simulink model "gm_sampleModel1956_3_sub_sub_sub"  (R2023a)
settings: Solver=VariableStepAuto  StartTime=0.0  StopTime=10.0  RelTol=1e-3
libraries: hdlsllib x4, simulink x3
settings Model: Creator=user1  LastModifiedBy=user1
settings OptimizationCC: BlockReduction=off  ConditionallyExecuteInputs=off
settings DebuggingCC: InheritedTsInSrcMsg=none

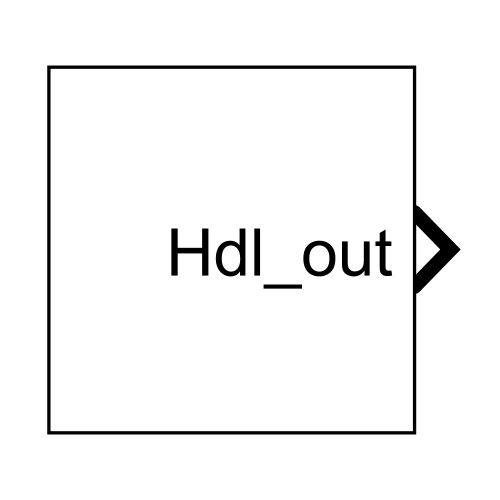
[thumbnail: Simulink's stored preview of the top-level diagram]
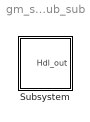
== system gm_sampleModel1956_3_sub_sub_sub ==
  Subsystem : Subsystem

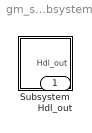
== system gm_sampleModel1956_3_sub_sub_sub/Subsystem ==
  Subsystem : Subsystem
  Hdl_out : Outport  OutDataTypeStr=uint8

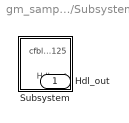
== system gm_sampleModel1956_3_sub_sub_sub/Subsystem/Subsystem ==
  Subsystem : Subsystem
  Hdl_out : Outport  OutDataTypeStr=uint8

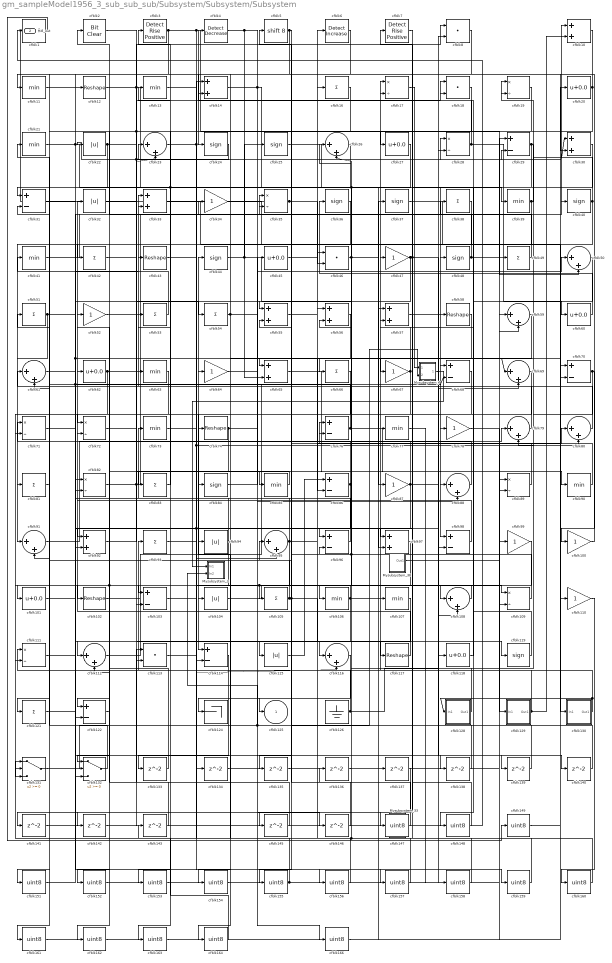
== system gm_sampleModel1956_3_sub_sub_sub/Subsystem/Subsystem/Subsystem ==
  Mysubsystem_3 : Subsystem  TreatAsAtomicUnit=on  RTWFcnName=Mysubsystem_3
      settings: RTWFcnNameOpts=User specified  RTWFileNameOpts=Use function name
  Mysubsystem_33 : Subsystem  TreatAsAtomicUnit=on  RTWFcnName=Mysubsystem_33
      settings: RTWFcnNameOpts=User specified  RTWFileNameOpts=Use function name
  Mysubsystem_38 : Subsystem  TreatAsAtomicUnit=on  RTWFcnName=Mysubsystem_38
      settings: RTWFcnNameOpts=User specified  RTWFileNameOpts=Use function name
  Mysubsystem_7 : Subsystem  TreatAsAtomicUnit=on  RTWFcnName=Mysubsystem_7
      settings: RTWFcnNameOpts=User specified  RTWFileNameOpts=Use function name
  cfblk1 : hdlsllib/Logic and Bit Operations/Compare To Zero  relop=<=  OutDataTypeStr=uint8
  cfblk{10,14,30,33,55..57,65,92,97} (10 alike) : Sum  OutDataTypeStr=uint8
  cfblk{34,47,52,64,67,78,87,99..100,110} (10 alike) : Gain  OutDataTypeStr=uint8
  cfblk{20,27,45,60,62,101,118} (7 alike) : Bias  Bias=0.0  SaturateOnIntegerOverflow=off
  cfblk{12,43,58,74,102,117} (6 alike) : Reshape
  cfblk{29,31,68,70,76,86,96,98,103,114,122} (11 alike) : Sum  Inputs=+-  OutDataTypeStr=uint8
  cfblk{22,32,94,104,115} (5 alike) : Abs  OutDataTypeStr=uint8  SaturateOnIntegerOverflow=off
  cfblk{16,38,42,49,51,53..54,66,81,83,93,105,121} (13 alike) : Sum  Inputs=+  OutDataTypeStr=uint8
  cfblk{11,13,21,39,41,63,73,77,85,90,106..107} (12 alike) : MinMax  OutDataTypeStr=uint8
  cfblk{23,26,50,59,61,69,79..80,88,91,95,108,112,116} (14 alike) : Sum  Inputs=|++  OutDataTypeStr=uint8
  cfblk{17,19,28,35,71..72,82,89,109,111} (10 alike) : Product  Inputs=*/  OutDataTypeStr=uint8  RndMeth=Zero  SaturateOnIntegerOverflow=on
  cfblk{8,18,46,113} (4 alike) : DotProduct  OutDataTypeStr=uint8
  cfblk{24..25,36..37,40,44,48,84,119} (9 alike) : Signum
  cfblk124 : Terminator
  cfblk126 : Ground
  cfblk128 : Subsystem
      settings: LibrarySourceBlock=|
      | hdlsllib/Ports &
      | Subsystems/Subsystem
  cfblk129 : Subsystem
      settings: LibrarySourceBlock=|
      | hdlsllib/Ports &
      | Subsystems/Subsystem
  cfblk130 : Subsystem
      settings: LibrarySourceBlock=|
      | hdlsllib/Ports &
      | Subsystems/Subsystem
  cfblk131 : Switch  OutDataTypeStr=uint8  SaturateOnIntegerOverflow=off  InputSameDT=off
  cfblk132 : Switch  OutDataTypeStr=uint8  SaturateOnIntegerOverflow=off  InputSameDT=off
  cfblk{133..143,145..146} (13 alike) : Delay  SampleTime=1
  cfblk{147..149,151..164,166} (18 alike) : DataTypeConversion  OutDataTypeStr=uint8  SaturateOnIntegerOverflow=off  RndMeth=Floor
  cfblk2 : simulink/Logic and Bit Operations/Bit Clear  iBit=0
      settings: LibrarySourceBlock=|
      | hdlsllib/Logic and Bit
      | Operations/Bit Clear
  cfblk3 : hdlsllib/Logic and Bit Operations/Detect Rise Positive  vinit=0  OutDataTypeStr=uint8
  cfblk4 : simulink/Logic and Bit Operations/Detect Decrease  vinit=0.0  OutDataTypeStr=uint8
      settings: LibrarySourceBlock=|
      | hdlsllib/Logic and Bit
      | Operations/Detect
      | Decrease
  cfblk5 : ArithShift  BitShiftNumber=8
  cfblk6 : simulink/Logic and Bit Operations/Detect Increase  vinit=0.0  OutDataTypeStr=uint8
      settings: LibrarySourceBlock=|
      | hdlsllib/Logic and Bit
      | Operations/Detect
      | Increase
  cfblk7 : hdlsllib/Logic and Bit Operations/Detect Rise Positive  vinit=0  OutDataTypeStr=uint8
  cfblk125 : Outport  OutDataTypeStr=uint8  VectorParamsAs1DForOutWhenUnconnected=off
  Hdl_out : Outport  Port=2  OutDataTypeStr=uint8
  wires:
  Mysubsystem_38/1(Out1) -> cfblk59/1
  Mysubsystem_33/1(Out1) -> cfblk1/1
  cfblk42/1 -> Mysubsystem_33/1(In1)
  Mysubsystem_7/1(Out1) -> Mysubsystem_3/1(In1)
  cfblk17/1 -> Mysubsystem_7/1(In1)
  cfblk166/1 -> cfblk59/2
  cfblk64/1 -> cfblk166/1
  cfblk164/1 -> cfblk143/1
  cfblk59/1 -> cfblk164/1
  cfblk163/1 -> cfblk99/1
  cfblk162/1 -> cfblk57/1
  cfblk99/1 -> cfblk162/1
  cfblk161/1 -> cfblk110/1
  cfblk160/1 -> cfblk94/1, cfblk26/1
  cfblk159/1 -> cfblk77/1
  cfblk13/1 -> cfblk159/1
  cfblk158/1 -> cfblk136/1, cfblk14/1
  cfblk157/1 -> cfblk56/2
  cfblk93/1 -> cfblk157/1
  cfblk156/1 -> cfblk56/1
  cfblk101/1 -> cfblk156/1
  cfblk155/1 -> cfblk131/1, cfblk118/1
  cfblk154/1 -> cfblk107/1
  cfblk153/1 -> cfblk29/1
  cfblk107/1 -> cfblk153/1
  cfblk152/1 -> cfblk137/1
  cfblk19/1 -> cfblk152/1
  cfblk151/1 -> cfblk92/2
  cfblk137/1 -> cfblk151/1
  cfblk149/1 -> cfblk20/1
  cfblk1/1 -> cfblk149/1
  cfblk148/1 -> cfblk7/1
  cfblk147/1 -> cfblk5/1
  cfblk7/1 -> cfblk147/1
  cfblk146/1 -> cfblk95/1
  cfblk145/1 -> cfblk112/2
  cfblk143/1 -> cfblk113/1
  cfblk142/1 -> cfblk8/2
  cfblk141/1 -> cfblk46/1
  cfblk140/1 -> cfblk55/2
  cfblk139/1 -> cfblk96/2
  cfblk138/1 -> cfblk76/2
  cfblk136/1 -> cfblk108/2
  cfblk135/1 -> cfblk35/2
  cfblk134/1 -> cfblk89/1
  cfblk103/1 -> cfblk134/1
  cfblk133/1 -> cfblk82/1
  cfblk114/1 -> cfblk133/1
  cfblk11/1 -> cfblk12/1
  cfblk111/1 -> cfblk43/1
  cfblk45/1 -> cfblk38/1
  cfblk40/1 -> cfblk122/1, cfblk19/2
  cfblk5/1 -> cfblk125/1, cfblk61/2
  cfblk53/1 -> cfblk41/1
  cfblk77/1 -> cfblk158/1
  cfblk31/1 -> cfblk54/1
  cfblk29/1 -> cfblk67/1, cfblk79/2
  cfblk86/1 -> cfblk13/1, cfblk135/1
  cfblk16/1 -> cfblk112/1
  cfblk18/1 -> cfblk103/1
  cfblk105/1 -> cfblk117/1, cfblk145/1, cfblk51/1
  cfblk26/1 -> cfblk42/1
  cfblk10/1 -> cfblk30/2
  cfblk35/1 -> cfblk46/2, Hdl_out/1
  cfblk52/1 -> cfblk6/1
  cfblk73/1 -> cfblk109/2, cfblk105/1
  cfblk55/1 -> cfblk16/1
  cfblk113/1 -> cfblk95/2
  cfblk109/1 -> cfblk61/1, cfblk26/2
  cfblk56/1 -> cfblk155/1
  cfblk22/1 -> cfblk101/1, cfblk8/1
  cfblk102/1 -> cfblk84/1
  cfblk104/1 -> cfblk109/1
  cfblk8/1 -> cfblk27/1
  cfblk132/1 -> cfblk21/1
  cfblk122/1 -> cfblk52/1
  cfblk118/1 -> cfblk18/1
  cfblk72/1 -> cfblk17/2
  cfblk89/1 -> cfblk76/1
  cfblk97/1 -> cfblk141/1, cfblk142/1
  cfblk116/1 -> cfblk124/1
  cfblk85/1 -> cfblk83/1
  cfblk106/1 -> cfblk40/1, cfblk104/1, cfblk132/2
  cfblk83/1 -> cfblk23/1
  cfblk61/1 -> cfblk68/2, cfblk138/1
  cfblk20/1 -> cfblk113/2, cfblk31/1, cfblk11/1
  cfblk4/1 -> cfblk65/2, cfblk146/1
  cfblk81/1 -> cfblk121/1
  cfblk94/1 -> cfblk73/1, cfblk131/3
  cfblk39/1 -> cfblk19/1, cfblk148/1
  cfblk126/1 -> cfblk111/1, cfblk28/2
  cfblk23/1 -> cfblk119/1, cfblk18/2
  cfblk46/1 -> cfblk96/1, cfblk70/2
  cfblk119/1 -> cfblk57/2
  cfblk58/1 -> cfblk86/2
  cfblk50/1 -> cfblk78/1
  cfblk27/1 -> cfblk161/1, cfblk163/1, cfblk66/1
  cfblk76/1 -> cfblk90/1, cfblk31/2
  cfblk47/1 -> cfblk97/1, cfblk140/1, cfblk103/2
  cfblk128/1(Out1) -> cfblk64/1
  cfblk92/1 -> cfblk29/2
  cfblk57/1 -> cfblk58/1
  cfblk49/1 -> cfblk2/1
  cfblk110/1 -> cfblk160/1
  cfblk74/1 -> cfblk92/1, cfblk88/2
  cfblk32/1 -> cfblk30/1, cfblk14/2
  cfblk25/1 -> cfblk87/1
  cfblk54/1 -> cfblk50/1, cfblk154/1
  cfblk63/1 -> cfblk91/2
  cfblk34/1 -> cfblk130/1(In1)
  cfblk121/1 -> cfblk82/2
  cfblk30/1 -> cfblk68/1
  cfblk37/1 -> cfblk70/1
  cfblk78/1 -> cfblk129/1(In1)
  cfblk2/1 -> cfblk85/1
  cfblk80/1 -> cfblk63/1
  cfblk36/1 -> cfblk55/1
  cfblk12/1 -> cfblk48/1, cfblk23/2
  cfblk90/1 -> cfblk35/1
  cfblk6/1 -> cfblk74/1
  cfblk112/1 -> cfblk37/1
  cfblk48/1 -> cfblk3/1, cfblk50/2
  cfblk91/1 -> cfblk79/1
  cfblk84/1 -> cfblk45/1
  cfblk24/1 -> cfblk22/1
  cfblk71/1 -> cfblk34/1
  cfblk3/1 -> cfblk116/2, cfblk80/2, cfblk49/1, cfblk132/3
  cfblk98/1 -> cfblk72/2
  cfblk87/1 -> cfblk114/2, cfblk122/2, cfblk53/1, cfblk69/2
  cfblk66/1 -> cfblk71/2
  cfblk41/1 -> cfblk33/2
  cfblk82/1 -> cfblk10/1, cfblk28/1, cfblk115/1
  cfblk43/1 -> cfblk89/2
  cfblk14/1 -> cfblk39/1, cfblk139/1
  cfblk33/1 -> cfblk88/1
  cfblk62/1 -> cfblk65/1, cfblk131/2
  cfblk95/1 -> cfblk62/1, cfblk111/2, cfblk80/1
  cfblk88/1 -> cfblk71/1
  cfblk69/1 -> cfblk72/1
  cfblk100/1 -> cfblk24/1
  cfblk108/1 -> cfblk102/1
  cfblk68/1 -> cfblk114/1
  cfblk96/1 -> cfblk44/1
  cfblk60/1 -> cfblk36/1
  cfblk130/1(Out1) -> cfblk47/1, cfblk128/1(In1)
  cfblk70/1 -> cfblk116/1, cfblk100/1
  cfblk117/1 -> cfblk32/1
  cfblk67/1 -> cfblk17/1, cfblk132/1
  cfblk79/1 -> cfblk33/1
  cfblk65/1 -> cfblk98/1
  cfblk131/1 -> Mysubsystem_7/2(In2), Mysubsystem_3/2(In2)
  cfblk28/1 -> cfblk60/1, cfblk4/1
  cfblk21/1 -> cfblk108/1, cfblk98/2
  cfblk38/1 -> cfblk81/1
  cfblk44/1 -> cfblk106/1, cfblk25/1
  cfblk51/1 -> cfblk69/1, cfblk97/2, cfblk91/1
  cfblk129/1(Out1) -> cfblk93/1, cfblk10/2
  cfblk115/1 -> cfblk86/1

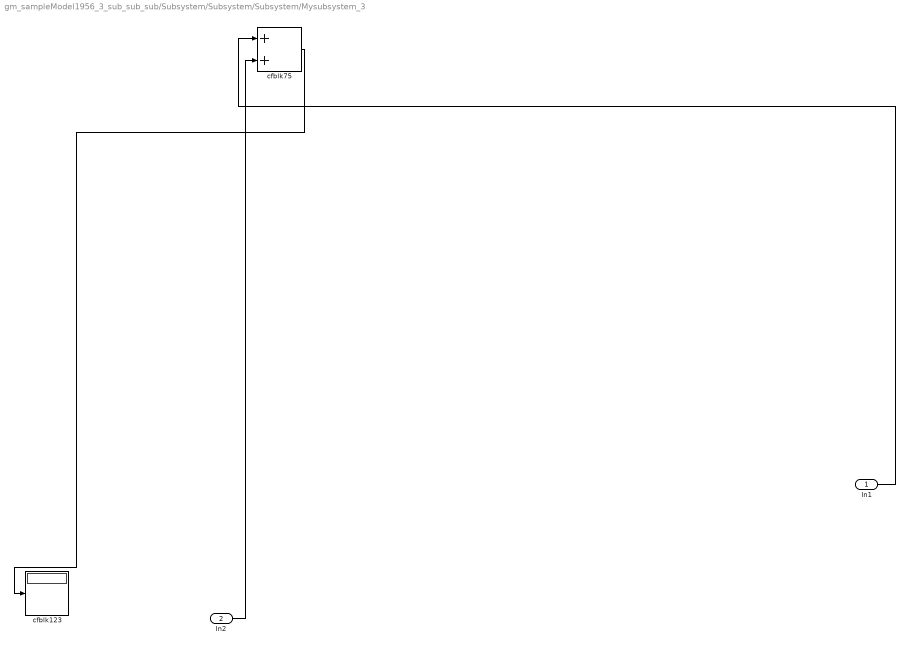
== system gm_sampleModel1956_3_sub_sub_sub/Subsystem/Subsystem/Subsystem/Mysubsystem_3 ==
  In1 : Inport
  In2 : Inport  Port=2
  cfblk123 : Display
  cfblk75 : Sum
  wires:
  cfblk75/1 -> cfblk123/1
  In2/1 -> cfblk75/2
  In1/1 -> cfblk75/1

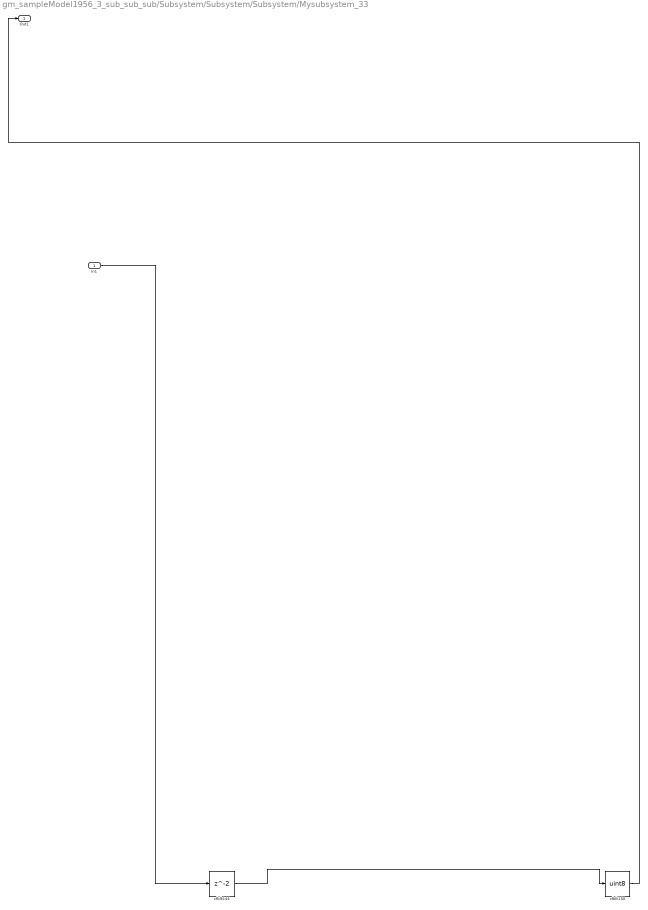
== system gm_sampleModel1956_3_sub_sub_sub/Subsystem/Subsystem/Subsystem/Mysubsystem_33 ==
  In1 : Inport
  cfblk144 : Delay  SampleTime=1
  cfblk150 : DataTypeConversion  OutDataTypeStr=uint8  SaturateOnIntegerOverflow=off  RndMeth=Floor
  Out1 : Outport
  wires:
  cfblk144/1 -> cfblk150/1
  In1/1 -> cfblk144/1
  cfblk150/1 -> Out1/1

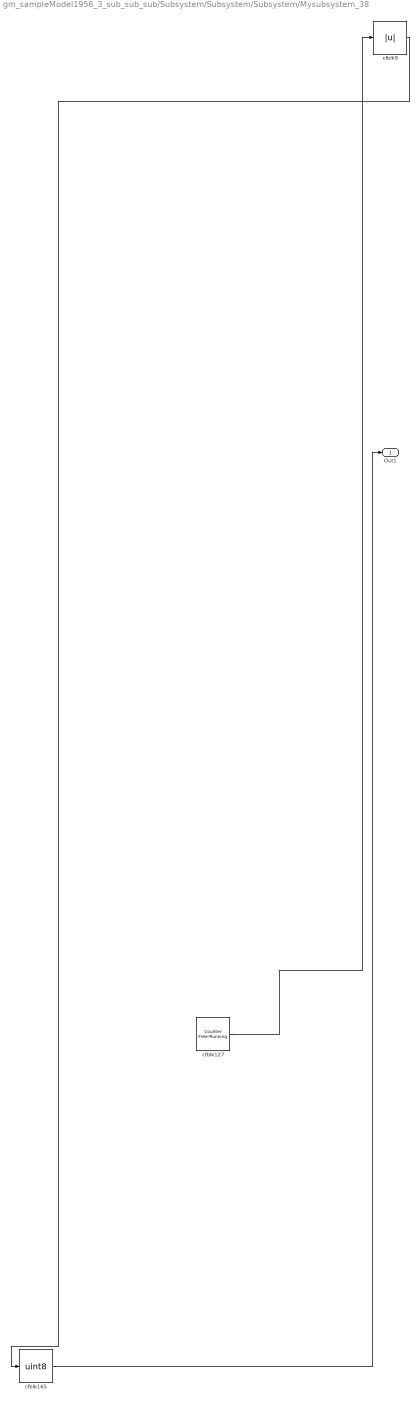
== system gm_sampleModel1956_3_sub_sub_sub/Subsystem/Subsystem/Subsystem/Mysubsystem_38 ==
  cfblk127 : hdlsllib/Sources/Counter Free-Running  NumBits=16  tsamp=-1
  cfblk165 : DataTypeConversion  OutDataTypeStr=uint8  SaturateOnIntegerOverflow=off  RndMeth=Floor
  cfblk9 : Abs  SaturateOnIntegerOverflow=off
  Out1 : Outport
  wires:
  cfblk165/1 -> Out1/1
  cfblk9/1 -> cfblk165/1
  cfblk127/1 -> cfblk9/1

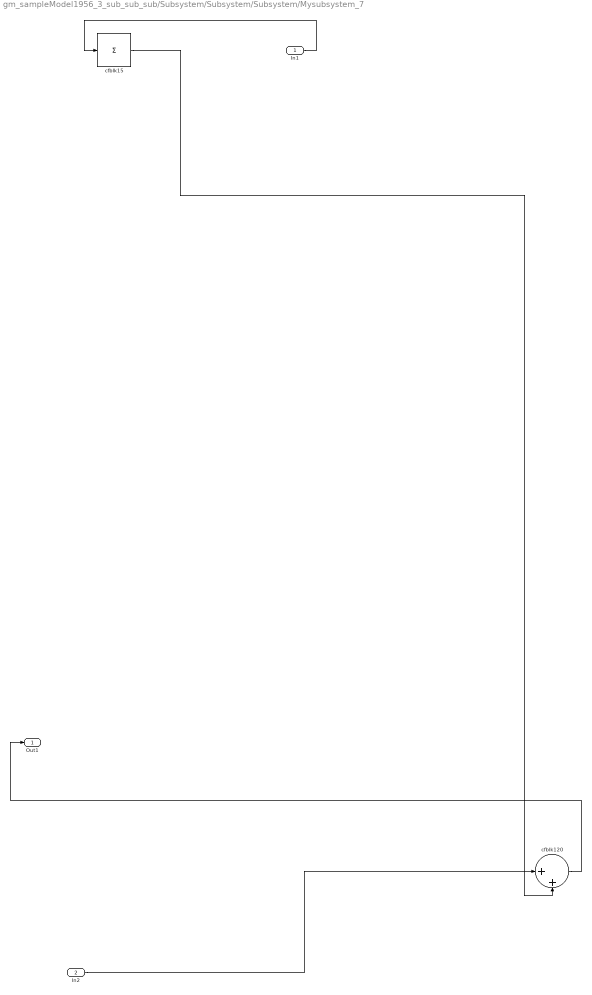
== system gm_sampleModel1956_3_sub_sub_sub/Subsystem/Subsystem/Subsystem/Mysubsystem_7 ==
  In1 : Inport
  In2 : Inport  Port=2
  cfblk120 : Sum  Inputs=|++
  cfblk15 : Sum  Inputs=+
  Out1 : Outport
  wires:
  cfblk15/1 -> cfblk120/2
  cfblk120/1 -> Out1/1
  In2/1 -> cfblk120/1
  In1/1 -> cfblk15/1

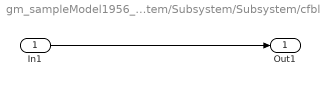
== system gm_sampleModel1956_3_sub_sub_sub/Subsystem/Subsystem/Subsystem/cfblk128 ==
  In1 : Inport
  Out1 : Outport
  wires:
  In1/1 -> Out1/1

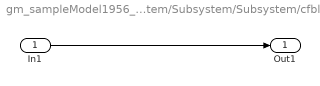
== system gm_sampleModel1956_3_sub_sub_sub/Subsystem/Subsystem/Subsystem/cfblk129 ==
  In1 : Inport
  Out1 : Outport
  wires:
  In1/1 -> Out1/1

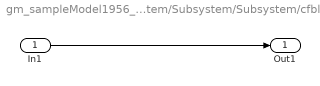
== system gm_sampleModel1956_3_sub_sub_sub/Subsystem/Subsystem/Subsystem/cfblk130 ==
  In1 : Inport
  Out1 : Outport
  wires:
  In1/1 -> Out1/1
